simulink model "simulazione"  (R2025b)
settings: Solver=ode45  StartTime=0.0  StopTime=15  RelTol=1e-6
values from neighbouring files (symbols this model uses):
  A = [ ... (first row only)    [codice_sintesi.m]
  B = [0; 1; 0; -1]    [codice_sintesi.m]
  C = [1 0 0 0; 0 0 1 0]    [codice_sintesi.m]
  Cs = [1 0 0 0]    [codice_sintesi.m]
  K = place(A,-B,v)    [codice_sintesi.m]
  L = Gamma - K * Pi    [codice_sintesi.m]
  PH = [ ... (first row only)    [codice_sintesi.m]
  Q = [0 -1 0]    [codice_sintesi.m]
  w = 0.1    [codice_sintesi.m]
settings Model: Creator=luca-callegari  LastModifiedBy=luca-callegari

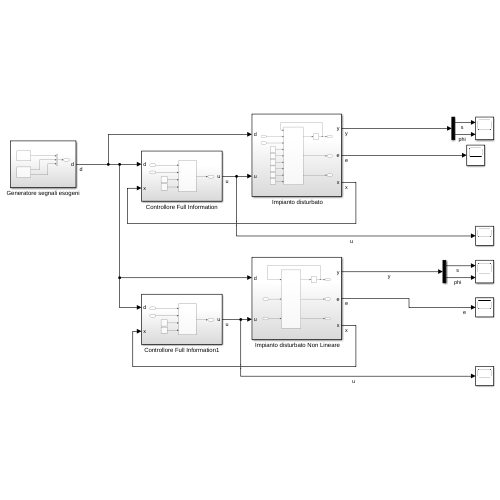
[thumbnail: Simulink's stored preview of the top-level diagram]
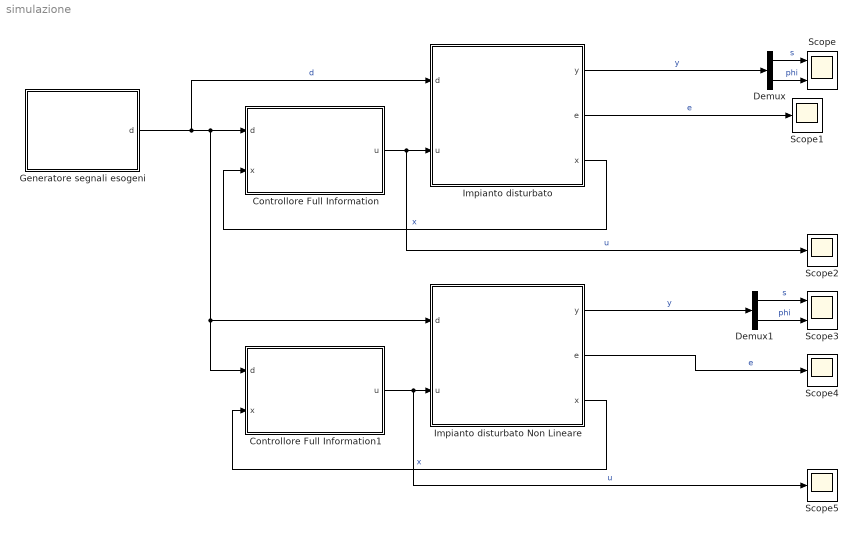
== system simulazione ==
  " Impianto disturbato" : Subsystem
  " Impianto disturbato Non Lineare" : Subsystem
  Controllore Full Information : Subsystem
  Controllore Full Information1 : Subsystem
  Demux : Demux  Outputs=2
  Demux1 : Demux  Outputs=2
  Generatore segnali esogeni : Subsystem
  Scope : Scope  NumInputPorts=2
      settings: ActiveDisplayYMinimum=-4.08613469526974  ActiveDisplayYMaximum=17.403217920025078  DataLoggingVariableName=ScopeData3
  Scope{1..2,4..5} (4 alike) : Scope
      Scope1 settings: ActiveDisplayYMinimum=-3.2809298670227611  ActiveDisplayYMaximum=16.21213792529214
      Scope2 settings: ActiveDisplayYMinimum=-135.79766357870963  ActiveDisplayYMaximum=154.7769429088346  DataLoggingVariableName=ScopeData2
      Scope4 settings: ActiveDisplayYMinimum=-952062.28477017349  ActiveDisplayYMaximum=8.5685472169173229E+6  DataLoggingVariableName=ScopeData5
      Scope5 settings: ActiveDisplayYMinimum=-1.242754738437545E+6  ActiveDisplayYMaximum=1.1184096829456028E+7  DataLoggingVariableName=ScopeData6
  Scope3 : Scope  NumInputPorts=2
      settings: ActiveDisplayYMinimum=-952062.85066808178  ActiveDisplayYMaximum=8.5685464854901172E+6  DataLoggingVariableName=ScopeData4
  wires:
  Controllore Full Information/1(u) -> Scope2/1, " Impianto disturbato"/2(u)  "u"
  " Impianto disturbato"/3(x) -> Controllore Full Information/2(x)  "x"
  " Impianto disturbato"/1(y) -> Demux/1  "y"
  Demux/1 -> Scope/1  "s"
  Demux/2 -> Scope/2  "phi"
  Generatore segnali esogeni/1(d) -> " Impianto disturbato"/1(d), " Impianto disturbato Non Lineare"/1(d), Controllore Full Information1/1(d), Controllore Full Information/1(d)  "d"
  " Impianto disturbato Non Lineare"/3(x) -> Controllore Full Information1/2(x)  "x"
  " Impianto disturbato"/2(e) -> Scope1/1  "e"
  Controllore Full Information1/1(u) -> Scope5/1, " Impianto disturbato Non Lineare"/2(u)  "u"
  " Impianto disturbato Non Lineare"/1(y) -> Demux1/1  "y"
  " Impianto disturbato Non Lineare"/2(e) -> Scope4/1  "e"
  Demux1/1 -> Scope3/1  "s"
  Demux1/2 -> Scope3/2  "phi"

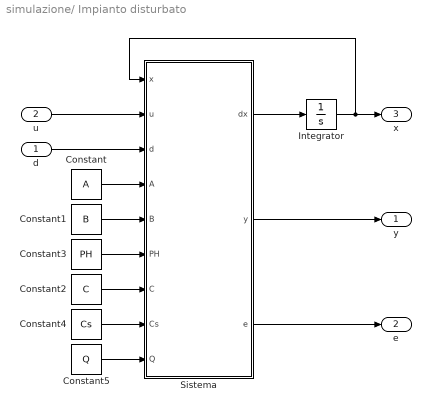
== system simulazione/ Impianto disturbato ==
  d : Inport
  u : Inport  Port=2
  Constant : Constant  Value=A  VectorParams1D=off
  Constant1 : Constant  Value=B  VectorParams1D=off
  Constant2 : Constant  Value=C  VectorParams1D=off
  Constant3 : Constant  Value=PH  VectorParams1D=off
  Constant4 : Constant  Value=Cs  VectorParams1D=off
  Constant5 : Constant  Value=Q  VectorParams1D=off
  Integrator : Integrator  InitialCondition=[0;0;0;0]
  Sistema : MATLAB Function  TreatAsAtomicUnit=on
  y : Outport
  e : Outport  Port=2
  x : Outport  Port=3
  wires:
  Sistema/1(dx) -> Integrator/1
  Integrator/1 -> Sistema/1(x), x/1
  Sistema/2(y) -> y/1
  u/1 -> Sistema/2(u)
  Constant/1 -> Sistema/4(A)
  Constant1/1 -> Sistema/5(B)
  Constant2/1 -> Sistema/7(C)
  d/1 -> Sistema/3(d)
  Constant3/1 -> Sistema/6(PH)
  Sistema/3(e) -> e/1
  Constant4/1 -> Sistema/8(Cs)
  Constant5/1 -> Sistema/9(Q)

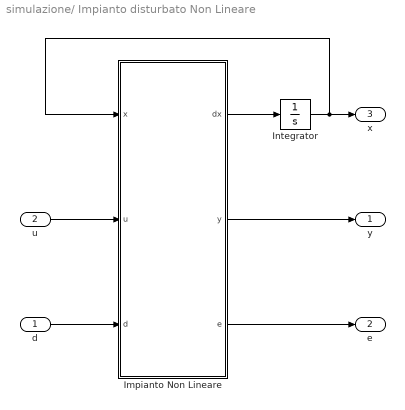
== system simulazione/ Impianto disturbato Non Lineare ==
  d : Inport
  u : Inport  Port=2
  Impianto Non Lineare : MATLAB Function  TreatAsAtomicUnit=on
  Integrator : Integrator  InitialCondition=[0;0;0;0]
  y : Outport
  e : Outport  Port=2
  x : Outport  Port=3
  wires:
  Impianto Non Lineare/1(dx) -> Integrator/1
  Integrator/1 -> Impianto Non Lineare/1(x), x/1
  Impianto Non Lineare/2(y) -> y/1
  u/1 -> Impianto Non Lineare/2(u)
  d/1 -> Impianto Non Lineare/3(d)
  Impianto Non Lineare/3(e) -> e/1

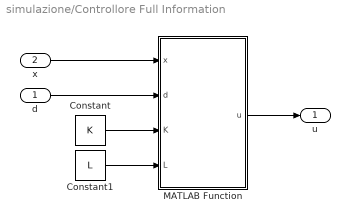
== system simulazione/Controllore Full Information ==
  d : Inport
  x : Inport  Port=2
  Constant : Constant  Value=K  VectorParams1D=off
  Constant1 : Constant  Value=L  VectorParams1D=off
  MATLAB Function : MATLAB Function  TreatAsAtomicUnit=on
  u : Outport
  wires:
  MATLAB Function/1(u) -> u/1
  x/1 -> MATLAB Function/1(x)
  d/1 -> MATLAB Function/2(d)
  Constant/1 -> MATLAB Function/3(K)
  Constant1/1 -> MATLAB Function/4(L)

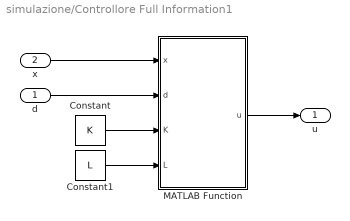
== system simulazione/Controllore Full Information1 ==
  d : Inport
  x : Inport  Port=2
  Constant : Constant  Value=K  VectorParams1D=off
  Constant1 : Constant  Value=L  VectorParams1D=off
  MATLAB Function : MATLAB Function  TreatAsAtomicUnit=on
  u : Outport
  wires:
  MATLAB Function/1(u) -> u/1
  x/1 -> MATLAB Function/1(x)
  d/1 -> MATLAB Function/2(d)
  Constant/1 -> MATLAB Function/3(K)
  Constant1/1 -> MATLAB Function/4(L)

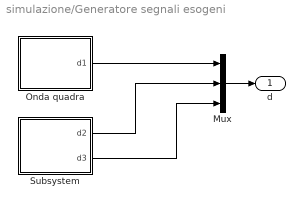
== system simulazione/Generatore segnali esogeni ==
  Mux : Mux  Inputs=3
  Onda quadra : Subsystem
  Subsystem : Subsystem
  d : Outport
  wires:
  Subsystem/1(d2) -> Mux/2
  Subsystem/2(d3) -> Mux/3
  Mux/1 -> d/1
  Onda quadra/1(d1) -> Mux/1

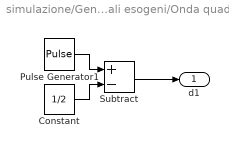
== system simulazione/Generatore segnali esogeni/Onda quadra ==
  Constant : Constant  Value=1/2
  Pulse Generator1 : DiscretePulseGenerator  PulseType=Time based  Period=50  PulseWidth=50
  Subtract : Sum  Inputs=+-
  d1 : Outport
  wires:
  Constant/1 -> Subtract/2
  Pulse Generator1/1 -> Subtract/1
  Subtract/1 -> d1/1

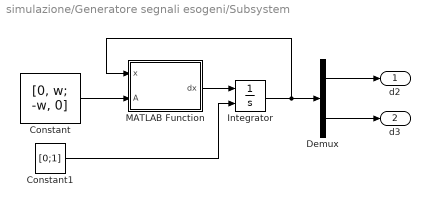
== system simulazione/Generatore segnali esogeni/Subsystem ==
  Constant : Constant  Value=[0, w; -w, 0]
  Constant1 : Constant  Value=[0;1]  VectorParams1D=off
  Demux : Demux  Outputs=2
  Integrator : Integrator  InitialConditionSource=external  InitialCondition=[1;0]
  MATLAB Function : MATLAB Function  TreatAsAtomicUnit=on
  d2 : Outport
  d3 : Outport  Port=2
  wires:
  Constant/1 -> MATLAB Function/2(A)
  MATLAB Function/1(dx) -> Integrator/1
  Integrator/1 -> MATLAB Function/1(x), Demux/1
  Demux/1 -> d2/1
  Demux/2 -> d3/1
  Constant1/1 -> Integrator/2

== matlab function simulazione/ Impianto disturbato/Sistema ==
  data: x input; dx output; u input; d input; y output; A input; B input; PH input; C input; Cs input; Q input; e output
function [dx, y, e] = fcn(x,u,d,A,B,PH,C,Cs,Q)
    dx = A*x + B*u + PH*d;
    y = C*x;
    e = Cs*x + Q*d;
end

== matlab function simulazione/Controllore Full Information/MATLAB Function ==
  data: x input; d input; K input; u output; L input
function u = fcn(x,d,K,L)
    u = K*x + L*d;
end

== matlab function simulazione/Generatore segnali esogeni/Subsystem/MATLAB Function ==
  data: x input; A input; dx output
function dx = fcn(x,A)
    dx = A*x;
end

== matlab function simulazione/ Impianto disturbato Non Lineare/Impianto Non Lineare ==
  data: x input; dx output; u input; d input; y output; e output
function [dx, y, e] = fcn(x,u,d)
    dx = zeros(4,1);
    dx(1) = x(2);
    dx(2) = -x(2) + u + d(1);
    dx(3) = x(4);
    dx(4) = 9.81*sin(x(3)) - dx(2)*cos(x(3));
    
    y = zeros(2,1);
    y(1) = x(1);
    y(2) = x(3);

    e = x(1) - d(2);
end

== matlab function simulazione/Controllore Full Information1/MATLAB Function ==
  data: x input; d input; K input; u output; L input
function u = fcn(x,d,K,L)
    u = K*x + L*d;
end
